simulink model "demo"  (R2015b)
settings: Solver=VariableStepAuto  StartTime=0.0  StopTime=10.0  RelTol=1e-3
settings Model: Creator=Administrator  LastModifiedBy=Administrator

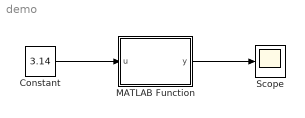
== system demo ==
  Constant : Constant  Value=3.14
  MATLAB Function : MATLAB Function  TreatAsAtomicUnit=on
  Scope : Scope
  wires:
  Constant/1 -> MATLAB Function/1(u)
  MATLAB Function/1(y) -> Scope/1

== matlab function demo/MATLAB Function ==
  data: u input; y output
function y = fcn(u)
%#codegen

y = sin(u*pi/180);
